simulink model "DcMotorwithequation"  (R2022a)
settings: Solver=VariableStepAuto  StartTime=0.0  StopTime=10.0  RelTol=1e-3
values from neighbouring files (symbols this model uses):
  b = 0.1    [DcCalculation.m]
  J = 0.01    [DcCalculation.m]
  Ke = 0.05    [DcCalculation.m]
  Kt = 0.05    [DcCalculation.m]
  L = 0.01    [DcCalculation.m]
  R = 1    [DcCalculation.m]
  V = 100    [DcCalculation.m]
libraries: slpidlib x1
settings Model: Creator=nivyachoudhary  LastModifiedBy=nivyachoudhary

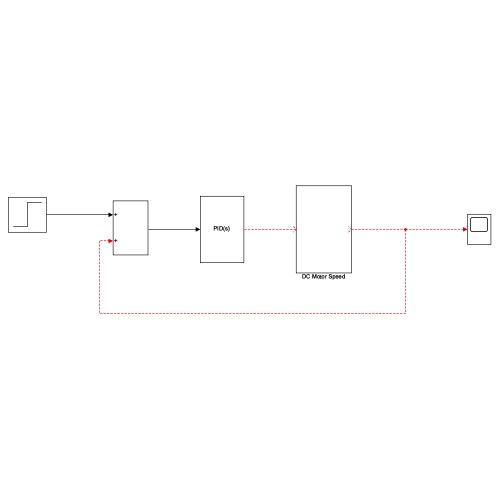
[thumbnail: Simulink's stored preview of the top-level diagram]
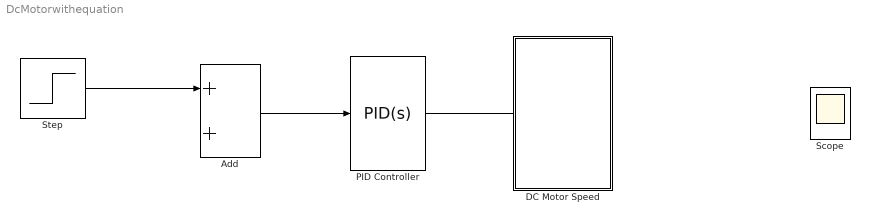
== system DcMotorwithequation ==
  Add : Sum
  DC Motor Speed : Subsystem
  PID Controller : slpidlib/PID Controller  Controller=PID  Form=Parallel  TimeDomain=Continuous-time  UseExternalTs=off  SampleTime=-1  IntegratorMethod=Forward Euler  FilterMethod=Forward Euler  ControllerParametersSource=internal  P=1  I=1  UseKiTs=off  D=0  N=100  UseFilter=on  TunerSelectOption=Transfer Function Based (PID Tuner App)  InitialConditionSource=internal  InitialConditionForIntegrator=0  InitialConditionForFilter=0  DifferentiatorICPrevScaledInput=0  ExternalReset=none  TrackingMode=off  Kt=1  LimitOutput=off  SatLimitsSource=internal  UpperSaturationLimit=inf  LowerSaturationLimit=-inf  LinearizeAsGain=on  AntiWindupMode=none  Kb=1  POutMin=[]  POutMax=[]  IOutMin=[]  IOutMax=[]  DOutMin=[]  DOutMax=[]  NOutMin=[]  NOutMax=[]  SumOutMin=[]  SumOutMax=[]  SaturationOutMin=[]  SaturationOutMax=[]  PParamMin=[]  PParamMax=[]  IParamMin=[]  IParamMax=[]  DParamMin=[]  DParamMax=[]  NParamMin=[]  NParamMax=[]  KbParamMin=[]  KbParamMax=[]  KtParamMin=[]  KtParamMax=[]  KbOutMin=[]  KbOutMax=[]  KtOutMin=[]  KtOutMax=[]  IntegratorOutMin=[]  IntegratorOutMax=[]  FilterOutMin=[]  FilterOutMax=[]  SumI1OutMin=[]  SumI1OutMax=[]  SumI2OutMin=[]  SumI2OutMax=[]  SumI3OutMin=[]  SumI3OutMax=[]  SumI4OutMin=[]  SumI4OutMax=[]  SumDOutMin=[]  SumDOutMax=[]  DifferentiatorOutMin=[]  DifferentiatorOutMax=[]  FilterDiffOutCoefMin=[]  FilterDiffOutCoefMax=[]  ReciprocalOutMin=[]  ReciprocalOutMax=[]  SumDenOutMin=[]  SumDenOutMax=[]  SumNumOutMin=[]  SumNumOutMax=[]  DivideOutMin=[]  DivideOutMax=[]  UdiffTsProdOutMin=[]  UdiffTsProdOutMax=[]  NTsProdOutMin=[]  NTsProdOutMax=[]  UintegralTsProdOutMin=[]  UintegralTsProdOutMax=[]  UngainTsProdOutMin=[]  UngainTsProdOutMax=[]  IntegratorContinuousStateAttributes=''  IntegratorStateMustResolveToSignalObject=off  IntegratorRTWStateStorageClass=Auto  FilterContinuousStateAttributes=''  FilterStateMustResolveToSignalObject=off  FilterRTWStateStorageClass=Auto  ParallelPVariant=InternalParameters  IdealPVariant=Disabled  IVariant=InternalParameters  DVariant=InternalParameters  IntegratorVariant=Continuous  SatVariant=Disabled  AWVariant=Passthrough  PCopyVariant=Disabled  TRVariant=Disabled  FdbkBlocksVariant=Forward  IdealPFdbkVariant=Disabled  SatFdbkVariant=Disabled  DerivativeFilterVariant=ContFilter  NVariant=InternalParameters  NCopyVariant=Disabled  FilterICVariant=InternalICsFilter  IntegratorICVariant=InternalICs  ExternalResetVariant=Disabled  TRSumVariant=Passthrough  SumFdbkVariant=Disabled  SumVariant=Sum_PID  TsampFilterVariant=InternalTs  TsampNgainVariant=Passthrough  TsampIntegralVariant=Passthrough  ExternalSaturationOutDataTypeStr=Inherit: Same as second input  aMode=0
  Scope : Scope
  Step : Step  Time=0  SampleTime=0
  wires:
  Add/1 -> PID Controller/1
  PID Controller/1 -> ?
  ? -> Add/2, Scope/1
  Step/1 -> Add/1

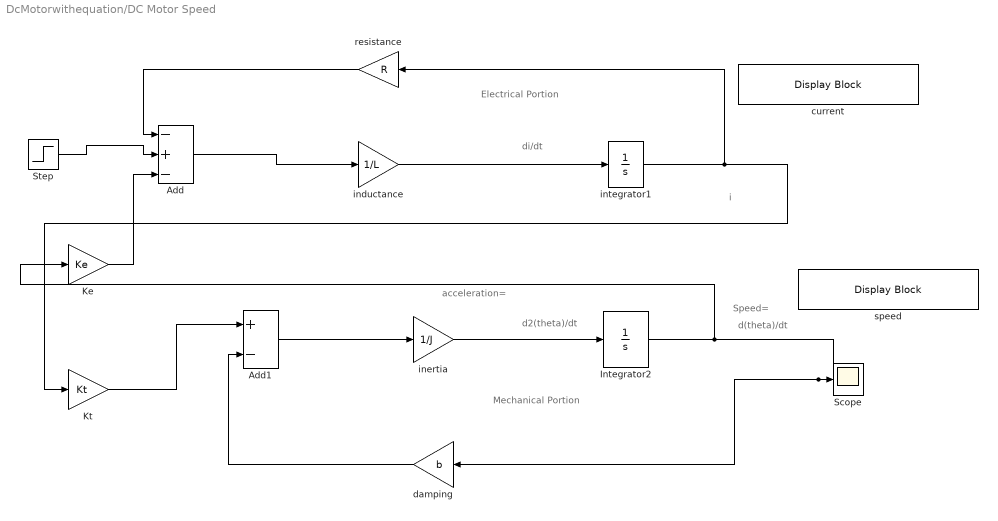
== system DcMotorwithequation/DC Motor Speed ==
  note: Speed=
  note: acceleration=
  note: Mechanical Portion
  note: Electrical Portion
  note: d(theta)/dt
  note: d2(theta)/dt
  note: di/dt
  note: i
  Add : Sum  Inputs=-+-
  Add1 : Sum  Inputs=+-
  Integrator2 : Integrator
  Ke : Gain  Gain=Ke
  Kt : Gain  Gain=Kt
  Scope : Scope
  Step : Step  Time=0  After=V  SampleTime=0
  current : DisplayBlock  LabelPosition=Hide  Transparency=1
  damping : Gain  Gain=b
  inductance : Gain  Gain=1/L
  inertia : Gain  Gain=1/J
  integrator1 : Integrator
  resistance : Gain  Gain=R
  speed : DisplayBlock  LabelPosition=Hide  Transparency=1
  wires:
  Kt/1 -> Add1/1
  Add/1 -> inductance/1
  integrator1/1 -> resistance/1, Kt/1
  inertia/1 -> Integrator2/1
  Integrator2/1 -> Ke/1, damping/1, Scope/1
  damping/1 -> Add1/2
  Add1/1 -> inertia/1
  Ke/1 -> Add/3
  inductance/1 -> integrator1/1
  resistance/1 -> Add/1
  Step/1 -> Add/2
